simulink model "schematic_diagram_3"  (R2022a)
settings: Solver=VariableStepAuto  StartTime=0.0  StopTime=10.0  RelTol=1e-3
settings Model: Creator=daixingze  LastModifiedBy=daixingze

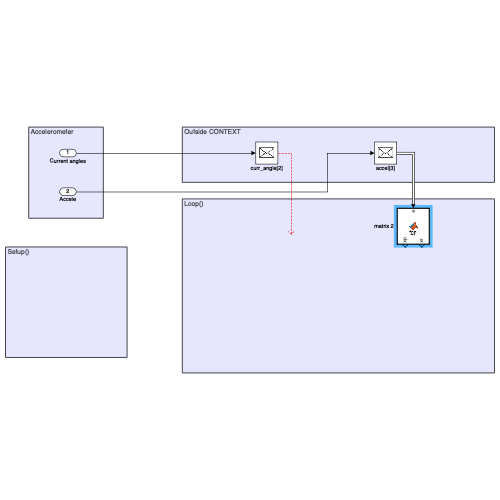
[thumbnail: Simulink's stored preview of the top-level diagram]
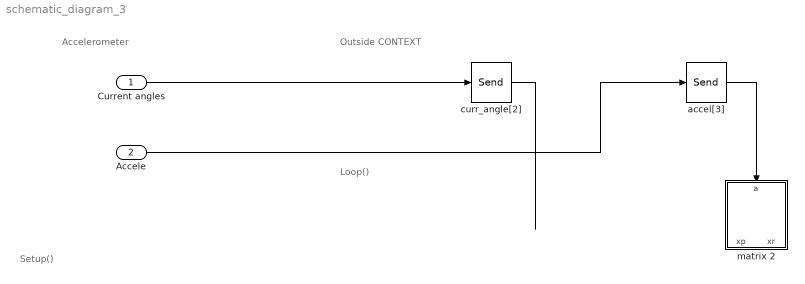
== system schematic_diagram_3 ==
  note: Loop()
  note: Setup()
  note: Accelerometer
  note: Outside CONTEXT
  Current angles : Inport
  Accele : Inport  Port=2
  accel[3] : Send  OutputPortMessageModes=m
  curr_angle[2] : Send  OutputPortMessageModes=m
  matrix 2 : MATLAB Function  TreatAsAtomicUnit=on
  wires:
  Current angles/1 -> curr_angle[2]/1
  Accele/1 -> accel[3]/1
  accel[3]/1 -> matrix 2/1(a)
  curr_angle[2]/1 -> ?

== matlab function schematic_diagram_3/matrix 2 ==
  data: a input; xp output; xr output
function [xp, xr] = fcn(a)
    R = 1;
    z1_error = -R*tan(xp);
    z2_error = (-sqrt(3)*sqrt(R^2+z1_error^2) / tan(xr) - z1_error) / 2;
    z3_error = -z1_error - z2_error;
